simulink library "simulink"  (Simulink 7.6)
settings: Solver=ode45  SolverMode=SingleTasking  StartTime=0.0  StopTime=10.0  RelTol=1e-3
PostLoadFcn:
  | setsysloc(bdroot)
undefined symbols (not defined in the file or in its folder): DiscIntNeverNeededParam, Floor, getdatatypespecs, NumBits1, NumBits2, sfunxy, sigbuilder_block, slcm, SlDemoSign, Slope1, Slope2
libraries: simulink x40, sl_helperblocks x2, eml_lib x1
(part 4 of 5)

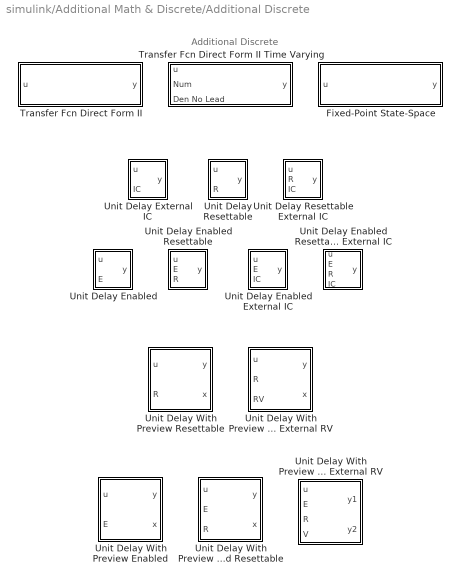
== system simulink/Additional Math & Discrete/Additional Discrete ==
  note: Additional Discrete
  Fixed-Point State-Space : Subsystem  mask(Fixed-Point State-Space){A=[2.6020 -2.2793 0.6708; 1 0 0; 0 1 0], B=[ 1; 0; 0], C=[0.0184    0.0024    0.0055], D=[0.0033], X0=0.0, InternalDataType=fixdt('double'), StateEqScaling=2^0, OutputEqScaling=2^0, LockScale=off, RndMeth=Floor, DoSatur=off}
      mask prompts: A "State Matrix A:"; B "Input Matrix B:"; C "Output Matrix C:"; D "Direct Feedthrough Matrix D:"; X0 "Initial condition for state:"; InternalDataType "Data type for internal calculations (e.g. fixdt(1, 16), fixdt('single')):"; StateEqScaling "Scaling for State Equation AX+BU (Slope, e.g. 2^-9):"; OutputEqScaling "Scaling for Output Equation CX+DU (Slope, e.g. 2^-9):"; LockScale "Lock output data type setting against changes by the fixed-point tools"; RndMeth "Integer rounding mode:"; DoSatur "Saturate to max or min when overflows occur"
      mask help: Discrete-time State-Space Realization
      mask init:
      | blkH = gcbh;
      | blkName = getfullname(blkH);
      | 
      | vRndMeth = get_param(blkH,'RndMeth');
      | vDoSatur = get_param(blkH,'DoSatur');
      | blks = {'State Matrix A','Input Matrix B','Output Matrix C','Direct Link Matrix D','Sum Output Equation','Sum State Equation','Downcast Next State X','Downcast Output Y'};
      | for i = 1:length(blks)
      |   set_param([blkName,'/',blks{i}],'RndMeth',vRndMeth, ...
      | 	  'DoSatur',vDoSatur);
      | end
      mask StyleString: edit,edit,edit,edit,edit,edit,edit,edit,checkbox,popup(Ceiling|Convergent|Floor|Nearest|Round|Simplest|Zero),checkbox
      mask TabNameString: Main,Main,Main,Main,Main,Signal Attributes,Signal Attributes,Signal Attributes,Signal Attributes,Signal Attributes,Signal Attributes
      mask Display:
      | text(0.5, 0.5, 'y(n)=Cx(n)+Du(n)', 'horizontalAlignment', 'center', 'verticalAlignment', 'bottom');
      | text(0.5, 0.5, 'x(n+1)=Ax(n)+Bu(n)', 'horizontalAlignment', 'center', 'verticalAlignment', 'top');
  Transfer Fcn Direct Form II : Subsystem  mask(Transfer Fcn Direct Form II){NumCoefVec=[0.2 0.3 0.2], DenCoefVec=[-0.9    0.6], vinit=0.0, RndMeth=Floor, DoSatur=off}
      mask prompts: NumCoefVec "Numerator coefficients:"; DenCoefVec "Denominator coefficients excluding lead (which must be 1.0):"; vinit "Initial condition:"; RndMeth "Integer rounding mode:"; DoSatur "Saturate to max or min when overflows occur"
      mask help:
      | A Direct Form II realization of the specified transfer function is used.  Only single input multiple output transfer functions are supported.
      |
      | The data types and scalings of the output, the coefficients, and any temporary variables are automatically selected.  The automatic choices will be acceptable in many situations.  In situations where the automatic choices give unacceptable results, manual layout of the filter is necessary.  For manual layout, it is suggested that the blocks under this mask be used as a starting point.
      |
      | Note 1:
      | The full denominator should have a leading coefficient of +1.0, but this leading coefficient should be excluded when entering the parameter.  For example, if the denominator is
      |   den =
      |             1         -1.7         0.72
      | just enter
      |   den(2:end)  =
      |          -1.7         0.72
      |
      | Note 2:
      | The numerator must be the same size as the full denominator.
      mask init:
      | blkH = gcbh;
      | blkName = getfullname(blkH);
      | 
      | vRndMeth = get_param(blkH,'RndMeth');
      | vDoSatur = get_param(blkH,'DoSatur');
      | DCGain = polyval(NumCoefVec,1)./polyval([1 DenCoefVec],1);
      | maxGain = max( 1, max(max(abs(DCGain))) );
      | maxGain = max( maxGain, abs(NumCoefVec(1)) );
      | OutputSlopeMult = 2^ceil(log2(maxGain));
      | DCGain = (1)./polyval([1 DenCoefVec],1);
      | maxGain = max( 1, max(max(abs(DCGain))) );
      | OutputSlopeMult2 = 2^ceil(log2(maxGain));
      | set_param([blkName,'/NumCoef'],'RndMeth',vRndMeth, ...
      | 	'DoSatur',vDoSatur);
      | set_param([blkName,'/DenCoef'],'RndMeth',vRndMeth, ...
      | 	'DoSatur',vDoSatur);
      | set_param([blkName,'/Downcast'],'RndMeth',vRndMeth, ...
      | 	'DoSatur',vDoSatur);
      | set_param([blkName,'/Downcast1'],'RndMeth',vRndMeth, ...
      | 	'DoSatur',vDoSatur);
      | set_param([blkName,'/Sum'],'RndMeth',vRndMeth, ...
      | 	'DoSatur',vDoSatur);
      mask StyleString: edit,edit,edit,popup(Ceiling|Convergent|Floor|Nearest|Round|Simplest|Zero),checkbox
      mask Display: dpoly(NumCoefVec,[1 DenCoefVec],'z-')
  Transfer Fcn Direct Form II Time Varying : Subsystem  mask(Transfer Fcn Direct Form II Time Varying){vinit=0.0, RndMeth=Floor, DoSatur=off}
      mask prompts: vinit "Initial condition:"; RndMeth "Integer rounding mode:"; DoSatur "Saturate to max or min when overflows occur"
      mask help:
      | A Direct Form II realization of the specified transfer function is used.  Only single input single output transfer functions are supported.
      |
      | The data types and scalings of the output, the coefficients, and any temporary variables are automatically selected.  The automatic choices will be acceptable in many situations.  In situations where the automatic choices give unacceptable results, manual layout of the filter is necessary.  For manual layout, it is suggested that the blocks under this mask be used as a starting point.
      |
      | Note 1:
      | The full denominator should have a leading coefficient of +1.0, but this leading coefficient should be excluded when entering the parameter.  For example, if the denominator is
      |   den =
      |             1         -1.7         0.72
      | just enter
      |   den(2:end)  =
      |          -1.7         0.72
      |
      | Note 2:
      | The numerator must be the same size as the full denominator.
      mask init:
      | blkH = gcbh;
      | blkName = getfullname(blkH);
      | 
      | vRndMeth = get_param(blkH,'RndMeth');
      | vDoSatur = get_param(blkH,'DoSatur');
      | set_param([blkName,'/Dot1'],'RndMeth',vRndMeth, ...
      | 	'DoSatur',vDoSatur);
      | set_param([blkName,'/Dot2'],'RndMeth',vRndMeth, ...
      | 	'DoSatur',vDoSatur);
      | set_param([blkName,'/Downcast'],'RndMeth',vRndMeth, ...
      | 	'DoSatur',vDoSatur);
      | set_param([blkName,'/Downcast1'],'RndMeth',vRndMeth, ...
      | 	'DoSatur',vDoSatur);
      | set_param([blkName,'/Sum'],'RndMeth',vRndMeth, ...
      | 	'DoSatur',vDoSatur);
      mask StyleString: edit,popup(Ceiling|Convergent|Floor|Nearest|Round|Simplest|Zero),checkbox
      mask Display: fprintf('Direct\nForm II')
  Unit Delay Enabled : Subsystem  mask(Unit Delay Enabled){vinit=0.0, tsamp=-1}
      mask prompts: vinit "Initial condition:"; tsamp "Sample time:"
      mask help:
      | Normally, the output is the signal u delayed by one sample period.
      | When the enable signal is false, the block is disabled, and the state and output values do not change.  The enable action is vectorized and supports scalar expansion.
      mask Display: dpoly(1,[1 0],'z')
  Unit Delay Enabled External IC : Subsystem  mask(Unit Delay Enabled External Initial Condition){tsamp=-1}
      mask prompts: tsamp "Sample time:"
      mask help:
      | Normally, the output is the signal u delayed by one sample period.
      | The initial condition is given by the signal IC.
      | When the enable signal is false, the block is disabled, and the state and output values do not change except for resets.  The enable action is vectorized and supports scalar expansion.
      mask Display: dpoly(1,[1 0],'z')
  Unit Delay Enabled Resettable : Subsystem  mask(Unit Delay Enabled Resettable){vinit=0.0, tsamp=-1}
      mask prompts: vinit "Initial condition:"; tsamp "Sample time:"
      mask help:
      | Normally, the output is the signal u delayed by one sample period.
      | When the reset signal R is true, the state and the output are always set equal to the initial condition parameter.  This reset action is vectorized and supports scalar expansion.
      | When the enable signal is false, the block is disabled, and the state and output values do not change except for resets.  The enable action is vectorized and supports scalar expansion.
      mask Display: dpoly(1,[1 0],'z')
  Unit Delay Enabled Resettable External IC : Subsystem  mask(Unit Delay Enabled Resettable External Initial Condition){tsamp=-1}
      mask prompts: tsamp "Sample time:"
      mask help:
      | Normally, the output is the signal u delayed by one sample period.
      | When the reset signal R is true, the state and the output are always set equal to the initial condition signal IC.  This reset action is vectorized and supports scalar expansion.
      | When the enable signal is false, the block is disabled, and the state and output values do not change except for resets.  The enable action is vectorized and supports scalar expansion.
      mask Display: dpoly(1,[1 0],'z')
  Unit Delay External IC : Subsystem  mask(Unit Delay External Initial Condition){tsamp=-1}
      mask prompts: tsamp "Sample time:"
      mask help:
      | Normally, the output is the signal u delayed by one sample period.
      | The initial condition is given by the signal IC.
      mask Display: dpoly(1,[1 0],'z')
  Unit Delay Resettable : Subsystem  mask(Unit Delay Resettable){vinit=0.0, tsamp=-1}
      mask prompts: vinit "Initial condition:"; tsamp "Sample time:"
      mask help:
      | Normally, the output is the signal u delayed by one sample period.
      | When the reset signal R is true, the state and the output are always set equal to the initial condition parameter.  This reset action is vectorized and supports scalar expansion.
      mask Display: dpoly(1,[1 0],'z')
  Unit Delay Resettable External IC : Subsystem  mask(Unit Delay Resettable External Initial Condition){tsamp=-1}
      mask prompts: tsamp "Sample time:"
      mask help:
      | Normally, the output is the signal u delayed by one sample period.
      | When the reset signal R is true, the state and the output are always set equal to the initial condition signal IC.  This reset action is vectorized and supports scalar expansion.
      mask Display: dpoly(1,[1 0],'z')
  Unit Delay With Preview Enabled : Subsystem  mask(Unit Delay With Preview Enabled){vinit=0.0, tsamp=-1}
      mask prompts: vinit "Initial condition:"; tsamp "Sample time:"
      mask help:
      | The Unit Delay With Preview Enabled normally has one output equal to the signal u, and a second output which is a unit-delayed version of the first output.
      |
      | When the enable signal is false, the block is disabled, and the state and output values do not change except during resets.
      mask Display:
      | plot([NaN 0.1 0.13 0.1 NaN 0.1 0.13 0.1 NaN 0.1 0.13 0.1 NaN -0.05 0.025 0.075 0.13 NaN -0.05 0.025 0.075 0.13 NaN 0.13 0.13 0.4475 0.4475 0.13 NaN 0.4475 0.4975 0.5525 0.5225 0.5525 0.5225 NaN 0.4475 0.4975 1.05 NaN 0.5525 0.5525 0.87 0.87 0.5525 NaN 0.71125 0.71125 NaN 0.6525 0.77 NaN 0.6525 0.77 0.6525 0.77 NaN 0.87 0.92 1.05 NaN 0.92 0.92 0.075 0.075 0.13],[NaN 0.846666666666667 0.816666666666667 0.786666666666667 NaN 0.58 0.55 0.52 NaN 0.313333333333333 0.283333333333333 0.253333333333333 NaN 0.75 0.75 0.816666666666667 0.816666666666667 NaN 0.25 0.25 0.55 0.55 NaN 0.15 0.95 0.95 0.15 0.15 NaN 0.55 0.35 0.35 0.38 0.35 0.32 NaN 0.55 0.75 0.75 NaN 0.15 0.55 0.55 0.15 0.15 NaN 0.5 0.4 NaN 0.35 0.35 NaN 0.3 0.3 0.2 0.2 NaN 0.35 0.25 0.25 NaN 0.25 0.05 0.05 0.283333333333333 0.283333333333333]);
      | text(0.23,0.806666666666667,'u');
      | text(0.23,0.54,'E');
  Unit Delay With Preview Enabled Resettable : Subsystem  mask(Unit Delay With Preview Enabled Resettable){vinit=0.0, tsamp=-1}
      mask prompts: vinit "Initial condition:"; tsamp "Sample time:"
      mask help:
      | The Unit Delay With Preview Enabled Resettable normally has one output equal to the signal u, and a second output which is a unit-delayed version of the first output.
      |
      | When the external reset signal R is true, the first output signal is forced to equal the initial condition. The second output signal is not affected until one time step later. The internal initial condition is also used to initialize the state when the model starts or when a parent enabled subsystem is reset.
      |
      | When the enable signal is false, the block is disabled, and the state and output values do not change except during resets.
      mask Display:
      | plot([NaN 0.1 0.13 0.1 NaN 0.1 0.13 0.1 NaN 0.1 0.13 0.1 NaN 0.1 0.13 0.1 NaN -0.05 0.025 0.075 0.13 NaN -0.05 0.025 0.075 0.13 NaN -0.05 0.025 0.075 0.13 NaN 0.13 0.13 0.4475 0.4475 0.13 NaN 0.4475 0.4975 0.5525 0.5225 0.5525 0.5225 NaN 0.4475 0.4975 1.05 NaN 0.5525 0.5525 0.87 0.87 0.5525 NaN 0.71125 0.71125 NaN 0.6525 0.77 NaN 0.6525 0.77 0.6525 0.77 NaN 0.87 0.92 1.05 NaN 0.92 0.92 0.075 0.075 0.13],[NaN 0.88 0.85 0.82 NaN 0.68 0.65 0.62 NaN 0.48 0.45 0.42 NaN 0.28 0.25 0.22 NaN 0.833333333333333 0.833333333333333 0.85 0.85 NaN 0.5 0.5 0.65 0.65 NaN 0.166666666666667 0.166666666666667 0.45 0.45 NaN 0.15 0.95 0.95 0.15 0.15 NaN 0.55 0.35 0.35 0.38 0.35 0.32 NaN 0.55 0.75 0.75 NaN 0.15 0.55 0.55 0.15 0.15 NaN 0.5 0.4 NaN 0.35 0.35 NaN 0.3 0.3 0.2 0.2 NaN 0.35 0.25 0.25 NaN 0.25 0.05 0.05 0.25 0.25]);
      | text(0.23,0.84,'u');
      | text(0.23,0.64,'E');
      | text(0.23,0.44,'R');
  Unit Delay With Preview Enabled Resettable External RV : Subsystem  mask(Unit Delay With Preview Enabled Resettable External RV){vinit=0.0, tsamp=-1}
      mask prompts: vinit "Initial condition:"; tsamp "Sample time:"
      mask help:
      | The Unit Delay With Preview Enabled Resettable External RV has both an external reset value RV and an internal initial condition. Normally, this block has one output equal to the signal u, and a second output which is a unit-delayed version of the first output.
      |
      | When the reset signal R is true, the first output signal is forced to equal RV. The second output signal is not affected until one time step later. The internal initial condition has a direct effect on the second output only when the model starts or when a parent enabled subsystem is reset.
      |
      | When the enable signal is false, the block is disabled, and the state and output values do not change except during resets.
      mask Display:
      | plot([NaN 0.1 0.13 0.1 NaN 0.1 0.13 0.1 NaN 0.1 0.13 0.1 NaN 0.1 0.13 0.1 NaN 0.1 0.13 0.1 NaN -0.05 0.025 0.075 0.13 NaN -0.05 0.025 0.075 0.13 NaN -0.05 0.025 0.075 0.13 NaN -0.05 0.025 0.075 0.13 NaN 0.13 0.13 0.4475 0.4475 0.13 NaN 0.4475 0.4975 0.5525 0.5225 0.5525 0.5225 NaN 0.4475 0.4975 1.05 NaN 0.5525 0.5525 0.87 0.87 0.5525 NaN 0.71125 0.71125 NaN 0.6525 0.77 NaN 0.6525 0.77 0.6525 0.77 NaN 0.87 0.92 1.05 NaN 0.92 0.92 0.075 0.075 0.13],[NaN 0.9 0.87 0.84 NaN 0.74 0.71 0.68 NaN 0.58 0.55 0.52 NaN 0.42 0.39 0.36 NaN 0.26 0.23 0.2 NaN 0.875 0.875 0.87 0.87 NaN 0.625 0.625 0.71 0.71 NaN 0.375 0.375 0.55 0.55 NaN 0.125 0.125 0.39 0.39 NaN 0.15 0.95 0.95 0.15 0.15 NaN 0.55 0.35 0.35 0.38 0.35 0.32 NaN 0.55 0.75 0.75 NaN 0.15 0.55 0.55 0.15 0.15 NaN 0.5 0.4 NaN 0.35 0.35 NaN 0.3 0.3 0.2 0.2 NaN 0.35 0.25 0.25 NaN 0.25 0.05 0.05 0.23 0.23]);
      | text(0.23,0.86,'u');
      | text(0.23,0.7,'E');
      | text(0.23,0.54,'R');
      | text(0.23,0.38,'RV');
  Unit Delay With Preview Resettable : Subsystem  mask(Unit Delay With Preview Resettable){vinit=0.0, tsamp=-1}
      mask prompts: vinit "Initial condition:"; tsamp "Sample time:"
      mask help:
      | The Unit Delay With Preview Resettable normally has one output equal to the signal u, and a second output which is a unit-delayed version of the first output.
      |
      | When the reset signal R is true, the first output signal is forced to equal the initial condition.  The second output signal is not affected until one time step later.  The internal initial condition is also used to initialize the state when the model starts or when a parent enabled subsystem is reset.
      mask Display:
      | plot([NaN 0.1 0.13 0.1 NaN 0.1 0.13 0.1 NaN -0.05 0.025 0.075 0.13 NaN -0.05 0.025 0.075 0.13 NaN 0.13 0.13 0.4475 0.4475 0.13 NaN 0.4475 0.4975 0.5525 0.5225 0.5525 0.5225 NaN 0.4475 0.4975 1.05 NaN 0.5525 0.5525 0.87 0.87 0.5525 NaN 0.71125 0.71125 NaN 0.6525 0.77 NaN 0.6525 0.77 0.6525 0.77 NaN 0.87 0.92 1.05],[NaN 0.755 0.725 0.695 NaN 0.305 0.275 0.245 NaN 0.75 0.75 0.725 0.725 NaN 0.25 0.25 0.275 0.275 NaN 0.0499999999999999 0.95 0.95 0.0499999999999999 0.0499999999999999 NaN 0.5 0.275 0.275 0.305 0.275 0.245 NaN 0.5 0.75 0.75 NaN 0.0499999999999999 0.5 0.5 0.0499999999999999 0.0499999999999999 NaN 0.45 0.325 NaN 0.275 0.275 NaN 0.225 0.225 0.0999999999999999 0.0999999999999999 NaN 0.275 0.25 0.25]);
      | text(0.23,0.715,'u');
      | text(0.23,0.265,'R');
  Unit Delay With Preview Resettable External RV : Subsystem  mask(Unit Delay With Preview Resettable External RV){vinit=0.0, tsamp=-1}
      mask prompts: vinit "Initial condition:"; tsamp "Sample time:"
      mask help:
      | The Unit Delay With Preview Resettable External RV has both an external reset value RV and an internal initial condition.  This block normally has one output equal to the signal u, and a second output which is a unit-delayed version of the first output.
      |
      | When the reset signal R is true, the first output signal is forced to equal RV. The second output signal is not affected until one time step later. The internal initial condition has a direct effect on the second output only when the model starts or when a parent enabled subsystem is reset.
      mask Display:
      | plot([NaN 0.1 0.13 0.1 NaN 0.1 0.13 0.1 NaN 0.1 0.13 0.1 NaN -0.05 0.025 0.075 0.13 NaN -0.05 0.025 0.075 0.13 NaN -0.05 0.025 0.075 0.13 NaN 0.13 0.13 0.4475 0.4475 0.13 NaN 0.4475 0.4975 0.5525 0.5225 0.5525 0.5225 NaN 0.4475 0.4975 1.05 NaN 0.5525 0.5525 0.87 0.87 0.5525 NaN 0.71125 0.71125 NaN 0.6525 0.77 NaN 0.6525 0.77 0.6525 0.77 NaN 0.87 0.92 1.05],[NaN 0.83 0.8 0.77 NaN 0.53 0.5 0.47 NaN 0.23 0.2 0.17 NaN 0.833333333333333 0.833333333333333 0.8 0.8 NaN 0.5 0.5 0.5 0.5 NaN 0.166666666666667 0.166666666666667 0.2 0.2 NaN 0.0499999999999999 0.95 0.95 0.0499999999999999 0.0499999999999999 NaN 0.5 0.275 0.275 0.305 0.275 0.245 NaN 0.5 0.75 0.75 NaN 0.0499999999999999 0.5 0.5 0.0499999999999999 0.0499999999999999 NaN 0.45 0.325 NaN 0.275 0.275 NaN 0.225 0.225 0.0999999999999999 0.0999999999999999 NaN 0.275 0.25 0.25]);
      | text(0.23,0.79,'u');
      | text(0.23,0.49,'R');
      | text(0.23,0.19,'RV');

== system simulink/Additional Math & Discrete/Additional Math: Increment - Decrement ==
  note: Increment/Decrement
  Decrement Real World : Subsystem
      mask Type: Real World Value Decrement
      mask Description:
      | Decrease the Real World Value of Signal by 1.0
      | Overflows will always wrap.
      mask Display: disp('V--')
  Decrement Stored Integer : Subsystem
      mask Type: Stored Integer Value Decrement
      mask Description:
      | Decrease the Stored Value of Signal by 1
      | Floating Point signals are decreased by 1.0
      | Overflows will always wrap.
      mask Display: disp('Q--')
  Decrement To Zero : Subsystem
      mask Type: Decrement To Zero
      mask Description:
      | Decrease the Real World Value of Signal by 1.0,
      | but never go below zero.
      mask Display: fprintf('max( V--, 0 )');
  Decrement Time To Zero : Subsystem
      mask Type: Decrement Time To Zero
      mask Description:
      | Decrease the Real World Value of Signal by the Sample Time Ts,
      | but never go below zero.
      | 
      | This block only works with fixed sample rates, so it will not work inside a triggered subsystem.
      mask Display: fprintf('max( V-Ts, 0 )');
  Increment Real World : Subsystem
      mask Type: Real World Value Increment
      mask Description:
      | Increase the Real World Value of Signal by 1.0
      | Overflows will always wrap.
      mask Display: disp('V++')
  Increment Stored Integer : Subsystem
      mask Type: Stored Integer Value Increment
      mask Description:
      | Increase the Stored Value of Signal by 1
      | Floating Point signals are increased by 1.0
      | Overflows will always wrap.
      mask Display: disp('Q++')

== system simulink/Commonly Used Blocks/Subsystem ==
  In1 : Inport
  Out1 : Outport
  wires:
  In1/1 -> Out1/1

== system simulink/Continuous/PID Controller ==
  u : Inport
  Derivative Gain : Gain  DisableCoverage=on  Gain=D  ParamMin=DParamMin  ParamMax=DParamMax  ParamDataTypeStr=DParamDataTypeStr  OutMin=DOutMin  OutMax=DOutMax  OutDataTypeStr=DOutDataTypeStr
  Filter : Integrator  DisableCoverage=on  InitialCondition=InitialConditionForFilter
  Filter Coefficient : Gain  DisableCoverage=on  Gain=N  ParamMin=NParamMin  ParamMax=NParamMax  ParamDataTypeStr=NParamDataTypeStr  OutMin=NOutMin  OutMax=NOutMax  OutDataTypeStr=NOutDataTypeStr
  Integral Gain : Gain  DisableCoverage=on  Gain=I  ParamMin=IParamMin  ParamMax=IParamMax  ParamDataTypeStr=IParamDataTypeStr  OutMin=IOutMin  OutMax=IOutMax  OutDataTypeStr=IOutDataTypeStr
  Integrator : Integrator  DisableCoverage=on  InitialCondition=InitialConditionForIntegrator
  Proportional Gain : Gain  DisableCoverage=on  Gain=P  ParamMin=PParamMin  ParamMax=PParamMax  ParamDataTypeStr=PParamDataTypeStr  OutMin=POutMin  OutMax=POutMax  OutDataTypeStr=POutDataTypeStr
  Sum : Sum  Inputs=+++  AccumDataTypeStr=SumAccumDataTypeStr  OutMin=SumOutMin  OutMax=SumOutMax  OutDataTypeStr=SumOutDataTypeStr
  SumD : Sum  DisableCoverage=on  Inputs=|+-  AccumDataTypeStr=SumDAccumDataTypeStr  OutMin=SumDOutMin  OutMax=SumDOutMax  OutDataTypeStr=SumDOutDataTypeStr
  y : Outport  InitialOutput=0
  wires:
  u/1 -> Proportional Gain/1, Integral Gain/1, Derivative Gain/1
  Proportional Gain/1 -> Sum/1
  Integral Gain/1 -> Integrator/1
  Derivative Gain/1 -> SumD/1
  SumD/1 -> Filter Coefficient/1
  Filter Coefficient/1 -> Filter/1, Sum/3
  Filter/1 -> SumD/2
  Integrator/1 -> Sum/2
  Sum/1 -> y/1

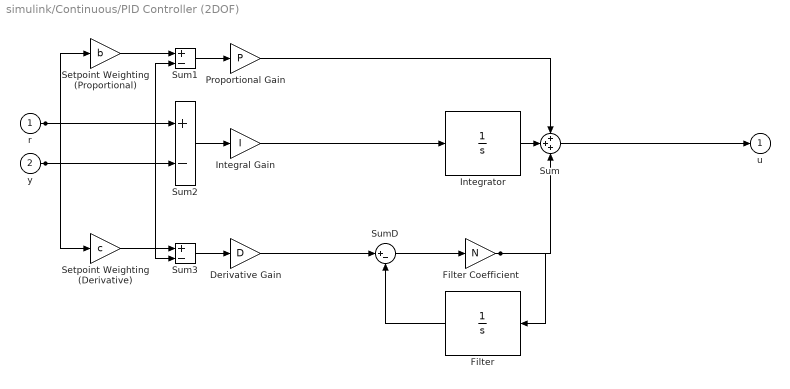
== system simulink/Continuous/PID Controller (2DOF) ==
  r : Inport
  y : Inport  Port=2
  Derivative Gain : Gain  DisableCoverage=on  Gain=D  ParamMin=DParamMin  ParamMax=DParamMax  ParamDataTypeStr=DParamDataTypeStr  OutMin=DOutMin  OutMax=DOutMax  OutDataTypeStr=DOutDataTypeStr
  Filter : Integrator  DisableCoverage=on  InitialCondition=InitialConditionForFilter
  Filter Coefficient : Gain  DisableCoverage=on  Gain=N  ParamMin=NParamMin  ParamMax=NParamMax  ParamDataTypeStr=NParamDataTypeStr  OutMin=NOutMin  OutMax=NOutMax  OutDataTypeStr=NOutDataTypeStr
  Integral Gain : Gain  DisableCoverage=on  Gain=I  ParamMin=IParamMin  ParamMax=IParamMax  ParamDataTypeStr=IParamDataTypeStr  OutMin=IOutMin  OutMax=IOutMax  OutDataTypeStr=IOutDataTypeStr
  Integrator : Integrator  DisableCoverage=on  InitialCondition=InitialConditionForIntegrator
  Proportional Gain : Gain  DisableCoverage=on  Gain=P  ParamMin=PParamMin  ParamMax=PParamMax  ParamDataTypeStr=PParamDataTypeStr  OutMin=POutMin  OutMax=POutMax  OutDataTypeStr=POutDataTypeStr
  Setpoint Weighting (Derivative) : Gain  DisableCoverage=on  Gain=c  ParamMin=cParamMin  ParamMax=cParamMax  ParamDataTypeStr=cParamDataTypeStr  OutMin=cOutMin  OutMax=cOutMax  OutDataTypeStr=cOutDataTypeStr
  Setpoint Weighting (Proportional) : Gain  DisableCoverage=on  Gain=b  ParamMin=bParamMin  ParamMax=bParamMax  ParamDataTypeStr=bParamDataTypeStr  OutMin=bOutMin  OutMax=bOutMax  OutDataTypeStr=bOutDataTypeStr
  Sum : Sum  Inputs=+++  AccumDataTypeStr=SumAccumDataTypeStr  OutMin=SumOutMin  OutMax=SumOutMax  OutDataTypeStr=SumOutDataTypeStr
  Sum1 : Sum  DisableCoverage=on  Inputs=+-  AccumDataTypeStr=Sum1AccumDataTypeStr  OutMin=Sum1OutMin  OutMax=Sum1OutMax  OutDataTypeStr=Sum1OutDataTypeStr
  Sum2 : Sum  DisableCoverage=on  Inputs=+-  AccumDataTypeStr=Sum2AccumDataTypeStr  OutMin=Sum2OutMin  OutMax=Sum2OutMax  OutDataTypeStr=Sum2OutDataTypeStr
  Sum3 : Sum  DisableCoverage=on  Inputs=+-  AccumDataTypeStr=Sum3AccumDataTypeStr  OutMin=Sum3OutMin  OutMax=Sum3OutMax  OutDataTypeStr=Sum3OutDataTypeStr
  SumD : Sum  DisableCoverage=on  Inputs=|+-  AccumDataTypeStr=SumDAccumDataTypeStr  OutMin=SumDOutMin  OutMax=SumDOutMax  OutDataTypeStr=SumDOutDataTypeStr
  u : Outport  InitialOutput=0
  wires:
  r/1 -> Setpoint Weighting (Proportional)/1, Setpoint Weighting (Derivative)/1, Sum2/1
  y/1 -> Sum1/2, Sum2/2, Sum3/2
  Setpoint Weighting (Proportional)/1 -> Sum1/1
  Setpoint Weighting (Derivative)/1 -> Sum3/1
  Sum1/1 -> Proportional Gain/1
  Sum2/1 -> Integral Gain/1
  Sum3/1 -> Derivative Gain/1
  Proportional Gain/1 -> Sum/1
  Integral Gain/1 -> Integrator/1
  Derivative Gain/1 -> SumD/1
  SumD/1 -> Filter Coefficient/1
  Filter Coefficient/1 -> Filter/1, Sum/3
  Filter/1 -> SumD/2
  Integrator/1 -> Sum/2
  Sum/1 -> u/1

== system simulink/Discontinuities/Coulomb & Viscous Friction ==
  u : Inport
  Gain : Gain  DisableCoverage=on  Gain=gain  SaturateOnIntegerOverflow=on  OutDataTypeStr=Inherit: Same as input
  Gain1 : Gain  DisableCoverage=on  Gain=offset  OutDataTypeStr=Inherit: Inherit via back propagation  SaturateOnIntegerOverflow=on
  Sign : Signum  DisableCoverage=on
  Sum : Sum  Inputs=|++  SaturateOnIntegerOverflow=on  InputSameDT=on  OutDataTypeStr=Inherit: Same as first input
  y : Outport
  wires:
  Sign/1 -> Gain1/1
  u/1 -> Gain/1, Sign/1
  Gain1/1 -> Sum/1
  Sum/1 -> y/1
  Gain/1 -> Sum/2

== system simulink/Discontinuities/Dead Zone Dynamic ==
  up : Inport
  u : Inport  Port=2
  lo : Inport  Port=3
  Diff : Sum  Inputs=+-  InputSameDT=on  OutDataTypeStr=Inherit: Same as first input
  Switch : Switch  Criteria=u2 ~= 0  ZeroCross=off  InputSameDT=on
  Switch1 : Switch  Criteria=u2 ~= 0  ZeroCross=off  InputSameDT=on
  u_GTE_up : RelationalOperator  DisableCoverage=on  OutDataTypeStr=boolean  ZeroCross=off
  u_GT_lo : RelationalOperator  DisableCoverage=on  Operator=>  OutDataTypeStr=boolean  ZeroCross=off
  y : Outport
  wires:
  Switch1/1 -> Switch/3
  u/1 -> u_GT_lo/1, Switch1/1, u_GTE_up/1, Diff/1
  u_GT_lo/1 -> Switch1/2
  Diff/1 -> y/1
  Switch/1 -> Diff/2
  lo/1 -> u_GT_lo/2, Switch1/3
  u_GTE_up/1 -> Switch/2
  up/1 -> u_GTE_up/2, Switch/1

== system simulink/Discontinuities/Rate Limiter Dynamic ==
  note: U(k)
  note: Y(k)
  up : Inport
  u : Inport  Port=2
  lo : Inport  Port=3
  Delay Input2 : UnitDelay  Description=Store in Global RAM  DisableCoverage=on  SampleTime=-1
  Difference Inputs1 : Sum  Description=Add in CPU  DisableCoverage=on  Inputs=+-  OutDataTypeStr=Inherit: Inherit via back propagation
  Difference Inputs2 : Sum  Description=Add in CPU  OutDataTypeStr=Inherit: Inherit via back propagation
  FixPt Data Type Duplicate : DataTypeDuplicate  DisableCoverage=on  NumInputPorts=7
  Saturation Dynamic : simulink/Discontinuities/Saturation Dynamic  SystemSampleTime=-1  OutMin=[]  OutMax=[]  OutDataTypeStr=Inherit: Same as second input  OutDataType=fixdt(1, 16)  OutScaling=2^-10  DoSatur=off
  delta fall limit : Product  DisableCoverage=on  Inputs=**  OutDataTypeStr=Inherit: Inherit via back propagation  SaturateOnIntegerOverflow=on
  delta rise limit : Product  DisableCoverage=on  Inputs=**  OutDataTypeStr=Inherit: Inherit via back propagation  SaturateOnIntegerOverflow=on
  sample time : SampleTimeMath  DisableCoverage=on  TsampMathOp=Ts Only  weightValue=1
  Y : Outport  InitialOutput=0
  wires:
  sample time/1 -> delta rise limit/2, delta fall limit/2
  lo/1 -> delta fall limit/1
  delta rise limit/1 -> Saturation Dynamic/1, FixPt Data Type Duplicate/6
  up/1 -> delta rise limit/1
  Difference Inputs2/1 -> FixPt Data Type Duplicate/1, Delay Input2/1, Y/1
  Delay Input2/1 -> FixPt Data Type Duplicate/2, Difference Inputs1/2, Difference Inputs2/2  "Y(k-1)"
  Saturation Dynamic/1 -> FixPt Data Type Duplicate/7, Difference Inputs2/1
  delta fall limit/1 -> Saturation Dynamic/3, FixPt Data Type Duplicate/3
  u/1 -> sample time/1, FixPt Data Type Duplicate/5, Difference Inputs1/1
  Difference Inputs1/1 -> Saturation Dynamic/2, FixPt Data Type Duplicate/4  "( U(k) - Y(k-1) )"

== system simulink/Discontinuities/Saturation Dynamic ==
  up : Inport
  u : Inport  Port=2
  lo : Inport  Port=3
  Data Type Duplicate : DataTypeDuplicate  DisableCoverage=on
  Data Type Propagation : simulink/Signal Attributes/Data Type Propagation  PropDataType=fixdt(1, 16)  IfRefDouble=double  IfRefSingle=single  IsSigned=IsSigned1  NumBitsBase=NumBits1  NumBitsMult=1  NumBitsAdd=0  NumBitsAllowFinal=1:128  PropScaling=2^-10  ValuesUsedBestPrec=[5 -7]  SlopeBase=Slope1  SlopeMult=1  SlopeAdd=0  BiasBase=Bias1  BiasMult=1  BiasAdd=0
  LowerRelop1 : RelationalOperator  DisableCoverage=on  Operator=>  OutDataTypeStr=boolean
  Switch : Switch  Criteria=u2 ~= 0  OutDataTypeStr=Inherit: Inherit via back propagation  ZeroCross=off
  Switch2 : Switch  Criteria=u2 ~= 0  OutMin=OutMin  OutMax=OutMax  OutDataTypeStr=Inherit: Inherit via back propagation  ZeroCross=off
  UpperRelop : RelationalOperator  DisableCoverage=on  Operator=<  OutDataTypeStr=boolean
  y : Outport  OutMin=OutMin  OutMax=OutMax
  wires:
  UpperRelop/1 -> Switch/2
  LowerRelop1/1 -> Switch2/2
  Switch2/1 -> y/1, Data Type Duplicate/1
  Switch/1 -> Data Type Propagation/3, Switch2/3, Data Type Duplicate/2
  lo/1 -> UpperRelop/2, Switch/1
  u/1 -> UpperRelop/1, Switch/3, LowerRelop1/1, Data Type Propagation/1, Data Type Propagation/2
  up/1 -> LowerRelop1/2, Switch2/1

== system simulink/Discontinuities/Wrap To Zero ==
  note: U(k)
  U : Inport
  Constant : Constant  DisableCoverage=on  Value=0  OutDataTypeStr=Inherit: Inherit via back propagation
  FixPt Data Type Duplicate1 : DataTypeDuplicate  DisableCoverage=on  NumInputPorts=3
  FixPt Switch : Switch  Criteria=u2 > Threshold  Threshold=Threshold  OutDataTypeStr=Inherit: Inherit via back propagation  ZeroCross=off
  Y : Outport  InitialOutput=0
  wires:
  Constant/1 -> FixPt Data Type Duplicate1/3, FixPt Switch/1
  FixPt Switch/1 -> Y/1, FixPt Data Type Duplicate1/1
  U/1 -> FixPt Data Type Duplicate1/2, FixPt Switch/3, FixPt Switch/2

== system simulink/Discrete/Difference ==
  note: U(k)
  note: ( U(k) - U(k-1) )
  U : Inport
  Diff : Sum  Description=Add in CPU  Inputs=+-  OutMin=OutMin  OutMax=OutMax  OutDataTypeStr=OutDataTypeStr
  UD : UnitDelay  Description=Store in Global RAM  DisableCoverage=on  X0=ICPrevInput  SampleTime=-1
  Y : Outport  OutMin=OutMin  OutMax=OutMax  InitialOutput=0
  wires:
  U/1 -> UD/1, Diff/1
  UD/1 -> Diff/2  "U(k-1)"
  Diff/1 -> Y/1

== system simulink/Discrete/Discrete Derivative ==
  note: U(k)
  note: ( U(k) - U(k-1) )
  U : Inport
  Data Type Duplicate : DataTypeDuplicate  DisableCoverage=on  NumInputPorts=3
  Diff : Sum  Description=Add in CPU  Inputs=+-  OutMin=OutMin  OutMax=OutMax  OutDataTypeStr=Inherit: Inherit via back propagation
  TSamp : SampleTimeMath  DisableCoverage=on  TsampMathOp=/  weightValue=inverseGainval  TsampMathImp=Offline Scaling Adjustment
  UD : UnitDelay  Description=Store in Global RAM  DisableCoverage=on  X0=ICPrevScaledInput  SampleTime=-1
  Y : Outport  OutMin=OutMin  OutMax=OutMax  InitialOutput=0
  wires:
  TSamp/1 -> Data Type Duplicate/2, Diff/1, UD/1
  Diff/1 -> Data Type Duplicate/1, Y/1
  UD/1 -> Data Type Duplicate/3, Diff/2  "U(k-1)"
  U/1 -> TSamp/1

== system simulink/Discrete/First-Order Hold ==
  u : Inport  OutDataTypeStr=double
  Clock : Clock
      settings: DisableCoverage=on  Decimation=10
  Digital Clock : DigitalClock  DisableCoverage=on  SampleTime=Ts
  Gain : Gain  DisableCoverage=on  Gain=1/Ts  SaturateOnIntegerOverflow=on  OutDataTypeStr=Inherit: Same as input  ParamDataTypeStr=Inherit: Same as input
  Hit  Crossing : HitCross  DisableCoverage=on  HitCrossingOffset=1  HitCrossingDirection=rising  ShowOutputPort=off
  Output : Sum  Inputs=++|  SaturateOnIntegerOverflow=on  InputSameDT=on  OutDataTypeStr=Inherit: Same as first input
  Product : Product  DisableCoverage=on  SaturateOnIntegerOverflow=on  InputSameDT=on  OutDataTypeStr=Inherit: Same as first input
  Sum : Sum  DisableCoverage=on  Inputs=|+-  SaturateOnIntegerOverflow=on  InputSameDT=on  OutDataTypeStr=Inherit: Same as first input
  Sum2 : Sum  DisableCoverage=on  Inputs=|+-  SaturateOnIntegerOverflow=on  InputSameDT=on  OutDataTypeStr=Inherit: Same as first input
  Unit Delay : UnitDelay  DisableCoverage=on  SampleTime=Ts
  Zero-Order Hold : ZeroOrderHold  DisableCoverage=on  SampleTime=Ts
  y : Outport  OutDataTypeStr=double
  wires:
  Sum/1 -> Product/1
  Unit Delay/1 -> Sum/2
  Product/1 -> Output/2
  Zero-Order Hold/1 -> Output/1, Sum/1
  u/1 -> Zero-Order Hold/1, Unit Delay/1
  Clock/1 -> Sum2/1
  Digital Clock/1 -> Sum2/2
  Gain/1 -> Hit  Crossing/1, Product/2
  Sum2/1 -> Gain/1
  Output/1 -> y/1

== system simulink/Discrete/Transfer Fcn First Order ==
  note: U(k)
  note: Y(k)
  U : Inport
  Data Type Duplicate : DataTypeDuplicate  DisableCoverage=on  NumInputPorts=3
  Diff : Sum  Description=Add in CPU  DisableCoverage=on  Inputs=+-
  Gain : Gain  DisableCoverage=on  Gain=PoleZ  OutDataTypeStr=Inherit: Inherit via back propagation
  Sum : Sum  Description=Add in CPU  OutDataTypeStr=Inherit: Inherit via back propagation
  UD : UnitDelay  Description=Store in Global RAM  DisableCoverage=on  X0=ICPrevOutput  SampleTime=-1
  Y : Outport  InitialOutput=0
  wires:
  Sum/1 -> Data Type Duplicate/1, UD/1, Y/1
  Gain/1 -> Data Type Duplicate/3, Sum/1  "(Pole) ( Y(k-1) - U(k) )"
  Diff/1 -> Gain/1  "( Y(k-1) - U(k) )"
  UD/1 -> Diff/1  "Y(k-1)"
  U/1 -> Data Type Duplicate/2, Sum/2, Diff/2

== system simulink/Discrete/Transfer Fcn Lead or Lag ==
  note: U(k)
  note: Y(k)
  u : Inport
  DataTypeProp : simulink/Signal Attributes/Data Type Propagation  PropDataType=fixdt(1, 16)  IfRefDouble=double  IfRefSingle=single  IsSigned=IsSigned1 or IsSigned2  NumBitsBase=max([NumBits1 NumBits2])  NumBitsMult=1  NumBitsAdd=0  NumBitsAllowFinal=1:128  PropScaling=2^-10  ValuesUsedBestPrec=[5 -7]  SlopeBase=min([Slope1 Slope2])  SlopeMult=OutputSlopeMult  SlopeAdd=0  BiasBase=Bias1  BiasMult=0  BiasAdd=0
  Delay Input : UnitDelay  Description=Store in Global RAM  DisableCoverage=on  X0=ICPrevInput  SampleTime=-1
      settings: AttributesFormatString=%<Description>
  Delay Output : UnitDelay  Description=Store in Global RAM  DisableCoverage=on  X0=ICPrevOutput  SampleTime=-1
      settings: AttributesFormatString=%<Description>
  Downcast : DataTypeConversion  Description=|  LockScale=on
      | Reduce from CPU Size
      |  to Global RAM Size
      settings: AttributesFormatString=%<Description>
  GainPole : Gain  Description=Multiply in CPU  DisableCoverage=on  Gain=PoleZ  LockScale=on
      settings: AttributesFormatString=%<Description>
  GainZero : Gain  Description=Multiply in CPU  DisableCoverage=on  Gain=ZeroZ  LockScale=on
      settings: AttributesFormatString=%<Description>
  Sum : Sum  Description=Add in CPU  DisableCoverage=on  Inputs=+-+  LockScale=on
      settings: AttributesFormatString=%<Description>
  y : Outport  InitialOutput=0
  wires:
  Downcast/1 -> DataTypeProp/3, Delay Output/1, y/1
  Sum/1 -> Downcast/1  "(Pole) Y(k-1) + U(k) - (Zero) U(k-1)"
  GainPole/1 -> Sum/3  "(Pole) Y(k-1)"
  GainZero/1 -> Sum/2  "(Zero) U(k-1)"
  Delay Input/1 -> GainZero/1  "U(k-1)"
  Delay Output/1 -> GainPole/1  "Y(k-1)"
  u/1 -> Delay Input/1, Sum/1, DataTypeProp/1, DataTypeProp/2

== system simulink/Discrete/Transfer Fcn Real Zero ==
  note: U(k)
  note: U(k) - (Zero) U(k-1)
  u : Inport
  DataTypeProp : simulink/Signal Attributes/Data Type Propagation  PropDataType=fixdt(1, 16)  IfRefDouble=double  IfRefSingle=single  IsSigned=IsSigned1 or IsSigned2  NumBitsBase=max([NumBits1 NumBits2])  NumBitsMult=1  NumBitsAdd=0  NumBitsAllowFinal=1:128  PropScaling=2^-10  ValuesUsedBestPrec=[5 -7]  SlopeBase=min([Slope1 Slope2])  SlopeMult=OutputSlopeMult  SlopeAdd=0  BiasBase=Bias1  BiasMult=0  BiasAdd=0
  Delay Input : UnitDelay  Description=Store in Global RAM  DisableCoverage=on  X0=ICPrevInput  SampleTime=-1
  GainZero : Gain  Description=Multiply in CPU  DisableCoverage=on  Gain=ZeroZ  LockScale=on
  Sum : Sum  Description=Add in CPU  Inputs=+-  OutDataTypeStr=Inherit: Inherit via back propagation  LockScale=on
  y : Outport  InitialOutput=0
  wires:
  u/1 -> DataTypeProp/2, DataTypeProp/1, Sum/1, Delay Input/1
  Delay Input/1 -> GainZero/1  "U(k-1)"
  GainZero/1 -> Sum/2  "(Zero) U(k-1)"
  Sum/1 -> y/1, DataTypeProp/3

== system simulink/Logic and Bit Operations/Bit Clear ==
  u : Inport
  FixPt Bitwise Operator3 : simulink/Logic and Bit Operations/Bitwise Operator  logicop=OR  UseBitMask=on  BitMask=2.^iBit  BitMaskRealWorld=Stored Integer
  FixPt Bitwise Operator4 : simulink/Logic and Bit Operations/Bitwise Operator  logicop=NOT  UseBitMask=off  BitMask=2^iBit  BitMaskRealWorld=Stored Integer
  FixPt Bitwise Operator5 : simulink/Logic and Bit Operations/Bitwise Operator  logicop=NOT  UseBitMask=off  BitMask=2^iBit  BitMaskRealWorld=Stored Integer
  y : Outport
  wires:
  FixPt Bitwise Operator3/1 -> FixPt Bitwise Operator5/1
  FixPt Bitwise Operator4/1 -> FixPt Bitwise Operator3/1
  u/1 -> FixPt Bitwise Operator4/1
  FixPt Bitwise Operator5/1 -> y/1

== system simulink/Logic and Bit Operations/Bit Set ==
  u : Inport
  FixPt Bitwise Operator1 : simulink/Logic and Bit Operations/Bitwise Operator  logicop=OR  UseBitMask=on  BitMask=2.^iBit  BitMaskRealWorld=Stored Integer
  y : Outport
  wires:
  FixPt Bitwise Operator1/1 -> y/1
  u/1 -> FixPt Bitwise Operator1/1

== system simulink/Logic and Bit Operations/Compare To Constant ==
  u : Inport
  Compare : RelationalOperator  Operator=<=  OutDataTypeStr=fixdt(0, 8)  InputSameDT=on
  Constant : Constant  DisableCoverage=on  Value=const  OutDataTypeStr=Inherit: Inherit via back propagation
  y : Outport
  wires:
  Compare/1 -> y/1
  Constant/1 -> Compare/2
  u/1 -> Compare/1

== system simulink/Logic and Bit Operations/Compare To Zero ==
  u : Inport
  Compare : RelationalOperator  Operator=<=  OutDataTypeStr=fixdt(0, 8)  InputSameDT=on
  Constant : Constant  DisableCoverage=on  Value=0  OutDataTypeStr=Inherit: Inherit via back propagation  PreserveConstantTs=on
  y : Outport
  wires:
  Compare/1 -> y/1
  u/1 -> Compare/1
  Constant/1 -> Compare/2

== system simulink/Logic and Bit Operations/Detect Change ==
  note: U(k)
  note: Edge
  U : Inport
  Delay Input1 : UnitDelay  Description=Store in Global RAM  DisableCoverage=on  X0=vinit  SampleTime=-1
  FixPt Relational Operator : RelationalOperator  Operator=~=  OutDataTypeStr=fixdt(0, 8)  ZeroCross=off
  Y : Outport  InitialOutput=0
  wires:
  U/1 -> Delay Input1/1, FixPt Relational Operator/1
  Delay Input1/1 -> FixPt Relational Operator/2  "U(k-1)"
  FixPt Relational Operator/1 -> Y/1

== system simulink/Logic and Bit Operations/Detect Decrease ==
  note: U(k)
  note: Edge
  U : Inport
  Delay Input1 : UnitDelay  Description=Store in Global RAM  DisableCoverage=on  X0=vinit  SampleTime=-1
  FixPt Relational Operator : RelationalOperator  Operator=<  OutDataTypeStr=fixdt(0, 8)  ZeroCross=off
  Y : Outport  InitialOutput=0
  wires:
  FixPt Relational Operator/1 -> Y/1
  Delay Input1/1 -> FixPt Relational Operator/2  "U(k-1)"
  U/1 -> FixPt Relational Operator/1, Delay Input1/1

== system simulink/Logic and Bit Operations/Detect Increase ==
  note: U(k)
  note: Edge
  U : Inport
  Delay Input1 : UnitDelay  Description=Store in Global RAM  DisableCoverage=on  X0=vinit  SampleTime=-1
  FixPt Relational Operator : RelationalOperator  Operator=>  OutDataTypeStr=fixdt(0, 8)  ZeroCross=off
  Y : Outport  InitialOutput=0
  wires:
  U/1 -> Delay Input1/1, FixPt Relational Operator/1
  Delay Input1/1 -> FixPt Relational Operator/2  "U(k-1)"
  FixPt Relational Operator/1 -> Y/1

== system simulink/Logic and Bit Operations/Detect Fall Negative ==
  note: U(k)
  note: Edge
  U : Inport
  Delay Input1 : UnitDelay  Description=Store in Global RAM  DisableCoverage=on  X0=vinit  SampleTime=-1
  FixPt Relational Operator : RelationalOperator  Operator=>  OutDataTypeStr=fixdt(0, 8)  ZeroCross=off
  Negative : simulink/Logic and Bit Operations/Compare To Zero  SystemSampleTime=-1  relop=<  LogicOutDataTypeMode=uint8  ZeroCross=off
  Y : Outport  InitialOutput=0
  wires:
  Negative/1 -> FixPt Relational Operator/1, Delay Input1/1  "U(k)"
  FixPt Relational Operator/1 -> Y/1
  Delay Input1/1 -> FixPt Relational Operator/2  "U(k-1)"
  U/1 -> Negative/1

== system simulink/Logic and Bit Operations/Detect Fall Nonpositive ==
  note: U(k)
  note: Edge
  U : Inport
  Delay Input1 : UnitDelay  Description=Store in Global RAM  DisableCoverage=on  X0=vinit  SampleTime=-1
  FixPt Relational Operator : RelationalOperator  Operator=>  OutDataTypeStr=fixdt(0, 8)  ZeroCross=off
  Nonpositive : simulink/Logic and Bit Operations/Compare To Zero  SystemSampleTime=-1  relop=<=  LogicOutDataTypeMode=uint8  ZeroCross=off
  Y : Outport  InitialOutput=0
  wires:
  U/1 -> Nonpositive/1
  Delay Input1/1 -> FixPt Relational Operator/2  "U(k-1)"
  FixPt Relational Operator/1 -> Y/1
  Nonpositive/1 -> Delay Input1/1, FixPt Relational Operator/1  "U(k)"

== system simulink/Logic and Bit Operations/Detect Rise Nonnegative ==
  note: U(k)
  note: Edge
  U : Inport
  Delay Input1 : UnitDelay  Description=Store in Global RAM  DisableCoverage=on  X0=vinit  SampleTime=-1
  FixPt Relational Operator : RelationalOperator  Operator=>  OutDataTypeStr=fixdt(0, 8)  ZeroCross=off
  Nonnegative : simulink/Logic and Bit Operations/Compare To Zero  SystemSampleTime=-1  relop=>=  LogicOutDataTypeMode=uint8  ZeroCross=off
  Y : Outport  InitialOutput=0
  wires:
  U/1 -> Nonnegative/1
  Delay Input1/1 -> FixPt Relational Operator/2  "U(k-1)"
  FixPt Relational Operator/1 -> Y/1
  Nonnegative/1 -> Delay Input1/1, FixPt Relational Operator/1  "U(k)"

== system simulink/Logic and Bit Operations/Detect Rise Positive ==
  note: U(k)
  note: Edge
  U : Inport
  Delay Input1 : UnitDelay  Description=Store in Global RAM  DisableCoverage=on  X0=vinit  SampleTime=-1
  FixPt Relational Operator : RelationalOperator  Operator=>  OutDataTypeStr=fixdt(0, 8)  ZeroCross=off
  Positive : simulink/Logic and Bit Operations/Compare To Zero  SystemSampleTime=-1  relop=>  LogicOutDataTypeMode=uint8  ZeroCross=off
  Y : Outport  InitialOutput=0
  wires:
  Positive/1 -> FixPt Relational Operator/1, Delay Input1/1  "U(k)"
  FixPt Relational Operator/1 -> Y/1
  Delay Input1/1 -> FixPt Relational Operator/2  "U(k-1)"
  U/1 -> Positive/1

== system simulink/Logic and Bit Operations/Extract Bits ==
  u : Inport
  DTProp1 : simulink/Signal Attributes/Data Type Propagation  PropDataType=fixdt(1, 16)  IfRefDouble=double  IfRefSingle=single  IsSigned=IsSigned1  NumBitsBase=NumBits1  NumBitsMult=0.5  NumBitsAdd=0  NumBitsAllowFinal=1:128  PropScaling=2^-10  ValuesUsedBestPrec=[5 -7]  SlopeBase=PosRange1  SlopeMult=2^0  SlopeAdd=0  BiasBase=Bias1  BiasMult=1  BiasAdd=0
  DTProp2 : simulink/Signal Attributes/Data Type Propagation  PropDataType=fixdt(1, 16)  IfRefDouble=double  IfRefSingle=single  IsSigned=IsSigned1  NumBitsBase=NumBits1  NumBitsMult=1  NumBitsAdd=0  NumBitsAllowFinal=1:128  PropScaling=1  ValuesUsedBestPrec=[5 -7]  SlopeBase=Slope1  SlopeMult=1  SlopeAdd=0  BiasBase=Bias1  BiasMult=1  BiasAdd=0
  Extract Desired Bits : DataTypeConversion  DisableCoverage=on
  Modify Scaling Only : DataTypeConversion  ConvertRealWorld=Stored Integer (SI)
  y : Outport
  wires:
  Extract Desired Bits/1 -> DTProp1/3, Modify Scaling Only/1, DTProp2/2, DTProp2/1
  u/1 -> DTProp1/1, DTProp1/2, Extract Desired Bits/1
  Modify Scaling Only/1 -> y/1, DTProp2/3

== system simulink/Logic and Bit Operations/Interval Test ==
  u : Inport
  AND : Logic  AllPortsSameDT=off  OutDataTypeStr=boolean
  FixPt Data Type Duplicate : DataTypeDuplicate  DisableCoverage=on  NumInputPorts=3
  Lower Limit : Constant  DisableCoverage=on  Value=lowlimit  OutDataTypeStr=Inherit: Inherit via back propagation
  Lower Test : RelationalOperator  DisableCoverage=on  Operator=<=  OutDataTypeStr=fixdt(0, 8)  ZeroCross=off
  Upper Limit : Constant  DisableCoverage=on  Value=uplimit  OutDataTypeStr=Inherit: Inherit via back propagation
  Upper Test : RelationalOperator  DisableCoverage=on  Operator=<=  OutDataTypeStr=fixdt(0, 8)  ZeroCross=off
  y : Outport
  wires:
  Lower Limit/1 -> Lower Test/1, FixPt Data Type Duplicate/2
  Upper Limit/1 -> Upper Test/2, FixPt Data Type Duplicate/3
  Lower Test/1 -> AND/1
  Upper Test/1 -> AND/2
  u/1 -> FixPt Data Type Duplicate/1, Lower Test/2, Upper Test/1
  AND/1 -> y/1

== system simulink/Logic and Bit Operations/Interval Test Dynamic ==
  up : Inport
  u : Inport  Port=2
  lo : Inport  Port=3
  FixPt Data Type Duplicate : DataTypeDuplicate  DisableCoverage=on  NumInputPorts=3
  FixPt Logical Operator : Logic  AllPortsSameDT=off  OutDataTypeStr=boolean
  Lower Test : RelationalOperator  DisableCoverage=on  Operator=<=  OutDataTypeStr=fixdt(0, 8)  ZeroCross=off
  Upper Test : RelationalOperator  DisableCoverage=on  Operator=<=  OutDataTypeStr=fixdt(0, 8)  ZeroCross=off
  y : Outport
  wires:
  FixPt Logical Operator/1 -> y/1
  u/1 -> Lower Test/2, Upper Test/1, FixPt Data Type Duplicate/2
  Upper Test/1 -> FixPt Logical Operator/2
  Lower Test/1 -> FixPt Logical Operator/1
  up/1 -> Upper Test/2, FixPt Data Type Duplicate/3
  lo/1 -> Lower Test/1, FixPt Data Type Duplicate/1

== system simulink/Logic and Bit Operations/Shift Arithmetic ==
  u : Inport
  shift : ArithShift  nBitShiftRight=nBitShiftRight  nBinPtShiftRight=nBinPtShiftRight
  y : Outport
  wires:
  u/1 -> shift/1
  shift/1 -> y/1

== system simulink/Lookup Tables/Cosine ==
  u : Inport
  Cosine : sl_helperblocks/Cosine  SystemSampleTime=-1  NumDataPoints=NumDataPoints  OutputWordLength=OutputWordLength
  cos(2*pi*u) : Outport
  wires:
  Cosine/1 -> cos(2*pi*u)/1
  u/1 -> Cosine/1

== system simulink/Lookup Tables/Sine ==
  u : Inport
  Sine : sl_helperblocks/Sine  SystemSampleTime=-1  NumDataPoints=NumDataPoints  OutputWordLength=OutputWordLength
  sin(2*pi*u) : Outport
  wires:
  Sine/1 -> sin(2*pi*u)/1
  u/1 -> Sine/1

== system simulink/Math Operations/Algebraic Constraint ==
  f(z) : Inport
  Initial Guess : InitialCondition  Value=z0
  Sum : Sum  DisableCoverage=on  Inputs=|++  SaturateOnIntegerOverflow=on  InputSameDT=on  OutDataTypeStr=Inherit: Same as first input
  z : Outport
  wires:
  f(z)/1 -> Sum/1
  Initial Guess/1 -> z/1, Sum/2
  Sum/1 -> Initial Guess/1

== system simulink/Math Operations/MinMax Running Resettable ==
  note: Reset
  u : Inport
  R : Inport  Port=2
  Data Type Duplicate : DataTypeDuplicate  DisableCoverage=on  NumInputPorts=3
  MinMax : MinMax  DisableCoverage=on  Inputs=2  OutDataTypeStr=Inherit: Inherit via back propagation  ZeroCross=off
      settings: LockScale=on
  Unit Delay With Preview Resettable : simulink/Additional Math & Discrete/Additional Discrete/Unit Delay With Preview Resettable  SystemSampleTime=-1  vinit=vinit  tsamp=-1
  y : Outport
  wires:
  Unit Delay With Preview Resettable/1 -> y/1
  MinMax/1 -> Data Type Duplicate/1, Unit Delay With Preview Resettable/1
  Unit Delay With Preview Resettable/2 -> Data Type Duplicate/2, MinMax/2
  u/1 -> Data Type Duplicate/3, MinMax/1
  R/1 -> Unit Delay With Preview Resettable/2

== system simulink/Math Operations/Slider Gain ==
  u : Inport
  Slider Gain : Gain  Gain=gain  SaturateOnIntegerOverflow=on  OutDataTypeStr=Inherit: Same as input  ParamDataTypeStr=Inherit: Same as input
  y : Outport
  wires:
  Slider Gain/1 -> y/1
  u/1 -> Slider Gain/1

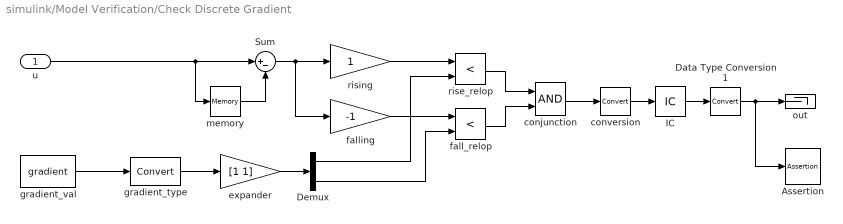
== system simulink/Model Verification/Check Discrete Gradient ==
  u : Inport
  Assertion : Assertion  DisableCoverage=on  Enabled=on
  Data Type Conversion1 : DataTypeConversion  DisableCoverage=on  SaturateOnIntegerOverflow=on  RndMeth=Zero
  Demux : Demux  DisableCoverage=on  Outputs=2
  IC : InitialCondition  DisableCoverage=on
  Sum : Sum  DisableCoverage=on  Inputs=|+-  SaturateOnIntegerOverflow=on  InputSameDT=on  OutDataTypeStr=Inherit: Same as first input
  conjunction : Logic  DisableCoverage=on
  conversion : DataTypeConversion  DisableCoverage=on  SaturateOnIntegerOverflow=on  RndMeth=Zero
  expander : Gain  DisableCoverage=on  Gain=[1 1]  SaturateOnIntegerOverflow=on  OutDataTypeStr=Inherit: Same as input  ParamDataTypeStr=Inherit: Same as input
  fall_relop : RelationalOperator  DisableCoverage=on  Operator=<  InputSameDT=on
  falling : Gain  DisableCoverage=on  Gain=-1  SaturateOnIntegerOverflow=on  OutDataTypeStr=Inherit: Same as input  ParamDataTypeStr=Inherit: Same as input
  gradient_type : DataTypeConversion  DisableCoverage=on  SaturateOnIntegerOverflow=on  RndMeth=Zero
  gradient_val : Constant  DisableCoverage=on  Value=gradient
  memory : Memory  DisableCoverage=on  InheritSampleTime=on
  out : Terminator
  rise_relop : RelationalOperator  DisableCoverage=on  Operator=<  InputSameDT=on
  rising : Gain  DisableCoverage=on  SaturateOnIntegerOverflow=on  OutDataTypeStr=Inherit: Same as input  ParamDataTypeStr=Inherit: Same as input
  wires:
  Data Type Conversion1/1 -> Assertion/1, out/1
  conversion/1 -> IC/1
  IC/1 -> Data Type Conversion1/1
  conjunction/1 -> conversion/1
  fall_relop/1 -> conjunction/2
  rise_relop/1 -> conjunction/1
  falling/1 -> fall_relop/1
  rising/1 -> rise_relop/1
  Sum/1 -> rising/1, falling/1
  memory/1 -> Sum/2
  Demux/2 -> fall_relop/2
  Demux/1 -> rise_relop/2
  expander/1 -> Demux/1
  u/1 -> Sum/1, memory/1
  gradient_val/1 -> gradient_type/1
  gradient_type/1 -> expander/1

== system simulink/Model Verification/Check  Dynamic Gap ==
  max : Inport
  min : Inport  Port=2
  u : Inport  Port=3
  Assertion : Assertion  DisableCoverage=on  Enabled=on
  disjunction : Logic  DisableCoverage=on  Operator=OR
  max_relop : RelationalOperator  DisableCoverage=on  Operator=<
  min_relop : RelationalOperator  DisableCoverage=on  Operator=<
  out : Terminator
  wires:
  max/1 -> max_relop/1
  min/1 -> min_relop/2
  u/1 -> min_relop/1, max_relop/2
  disjunction/1 -> Assertion/1, out/1
  min_relop/1 -> disjunction/2
  max_relop/1 -> disjunction/1
